simulink model "IPMSM_velocity_control"  (R2020b)
settings: Solver=FixedStepDiscrete  StartTime=0.0  StopTime=300e-3  FixedStep=Ts  RelTol=1e-3
PreLoadFcn:
  | ee_ipmsm_torque_based_load_control_data;
StopFcn:
  | ee_addSimlogTimeStamp(bdroot)
values from neighbouring files (symbols this model uses):
  K_aw = 100    [ee_ipmsm_torque_based_load_control_data.m]
  K_i = 200    [ee_ipmsm_torque_based_load_control_data.m]
  K_p = 1    [ee_ipmsm_torque_based_load_control_data.m]
  K_v = 1    [ee_ipmsm_torque_based_load_control_data.m]
  Ld = 0.00024368    [ee_ipmsm_torque_based_load_control_data.m]
  Lq = 0.00029758    [ee_ipmsm_torque_based_load_control_data.m]
  msg_period = 10e-3    (= 0.01)    [ee_ipmsm_torque_based_load_control_data.m]
  p = 5    [ee_ipmsm_torque_based_load_control_data.m]
  psim = 0.04366    [ee_ipmsm_torque_based_load_control_data.m]
  Ts = 5e-6    (= 5e-06)    [ee_ipmsm_torque_based_load_control_data.m]
undefined symbols (not defined in the file or in its folder): DiscIntNeverNeededParam, m, n, VDC_VECT
libraries: fl_lib x12, nesl_utility x12, ee_lib x5, fl_ps_legacy_lib x4, simulink x2, eeTransforms x2, slrealtimeutilitieslib x2, slrealtimeiplib x2, eePmsmCurrentController x1, eePmsmCurrentReferenceGen x1, eePmsmTorqueEstimator x1, eePwmGeneratorTwoLevel x1
CloseFcn:
  | try,close(h1_ee_ipmsm_torque_based_load_control),end
  | clear h1_ee_ipmsm_torque_based_load_control
  | 
  | clear simlog_ee_ipmsm_torque_based_load_control
  | clear logsout_ee_ipmsm_torque_based_load_control
Description:
  | IPMSM Torque-Based Load Control
settings Model: SimulationMode=accelerator  Creator=The MathWorks, Inc.  LastModifiedBy=Cliente
settings DataIOCC: MaxDataPoints=210000  ReturnWorkspaceOutputs=off  SignalLoggingName=logsout_ee_ipmsm_torque_based_load_control
settings OptimizationCC: DefaultParameterBehavior=Inlined  EnhancedBackFolding=on  PassReuseOutputArgsAs=Individual arguments  ZeroExternalMemoryAtStartup=off  ZeroInternalMemoryAtStartup=off  OptimizeBlockOrder=speed  DifferentSizesBufferReuse=on  OptimizationCustomize=off  EfficientTunableParamExpr=on
settings DebuggingCC: UnderspecifiedInitializationDetection=Classic  MergeDetectMultiDrivingBlocksExec=none  ParameterTunabilityLossMsg=error  SFUnexpectedBacktrackingDiag=warning  SFNoUnconditionalDefaultTransitionDiag=warning  SFExecutionAtInitializationDiag=none  ArithmeticOperatorsInVariantConditions=warning
settings SFSimCC: SimUseLocalCustomCode=off  MATLABDynamicMemAlloc=off  CustomCodeUndefinedFunction=UseInterfaceOnly
settings RTWCC: Description=Embedded Coder  SystemTargetFile=ert.tlc  TemplateMakefile=ert_default_tmf  RTWUseLocalCustomCode=off
settings CodeAppCC: ForceParamTrailComments=on  IgnoreCustomStorageClasses=off  OperatorAnnotations=on  SimulinkDataObjDesc=on  SFDataObjDesc=on  InsertBlockDesc=on
settings ERTTargetCC: GenerateSampleERTMain=on  InlinedParameterPlacement=NonHierarchical  ERTCustomFileTemplate=example_file_process.tlc
settings ConfigComp: CovMetricSettings=dw  CovSaveCumulativeToWorkspaceVar=on  CovSaveSingleToWorkspaceVar=on  CovExternalEMLEnable=off
settings SimscapeCC: SimscapeNormalizeSystem=off  SimscapeLogSimulationStatistics=on  SimscapeLogName=simlog_ee_ipmsm_torque_based_load_control  SimscapeLogDataHistory=210000

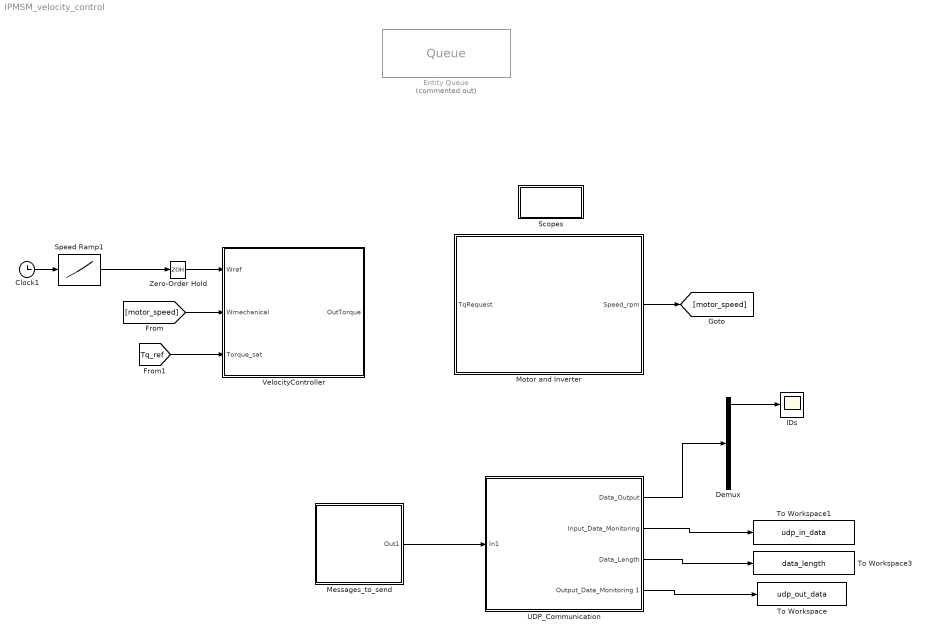
== system IPMSM_velocity_control ==
  Clock1 : Clock
  Demux : Demux  Outputs=5
  Entity Queue : Queue  Commented=on  InputPortMessageModes=m  OutputPortMessageModes=n,m  AverageWait=on
      settings: OutputPortMap=o2,o5
  IDs : Scope
  Messages_to_send : Subsystem
  Motor and Inverter : Subsystem
  Scopes : Subsystem
  Speed Ramp1 : Lookup_n-D  NumberOfTableDimensions=1  BreakpointsForDimension1=[0 .2 2]  Table=[0 200 200]  InternalRulePriority=Speed  RndMeth=Simplest  InputSameDT=on
  To Workspace : ToWorkspace  VariableName=udp_out_data  SaveFormat=Timeseries  SampleTime=-1
      settings: Save2DSignal=2-D array (concatenate along first dimension)
  To Workspace1 : ToWorkspace  VariableName=udp_in_data  SaveFormat=Timeseries  SampleTime=-1
      settings: Save2DSignal=2-D array (concatenate along first dimension)
  To Workspace3 : ToWorkspace  VariableName=data_length  SaveFormat=Timeseries  SampleTime=-1
      settings: Save2DSignal=2-D array (concatenate along first dimension)
  UDP_Communication : Subsystem
  VelocityController : Subsystem
  Zero-Order Hold : ZeroOrderHold  SampleTime=10e-3
  wires:
  Motor and Inverter/1(Speed_rpm) -> [motor_speed]
  Clock1/1 -> Speed Ramp1/1
  [Tq_ref] -> VelocityController/3(Torque_sat)
  Zero-Order Hold/1 -> VelocityController/1(Wref)
  Speed Ramp1/1 -> Zero-Order Hold/1
  Demux/1 -> IDs/1
  UDP_Communication/4(Output_Data_Monitoring 1) -> To Workspace/1
  UDP_Communication/2("Input_Data_Monitoring ") -> To Workspace1/1
  UDP_Communication/3(Data_Length) -> To Workspace3/1
  UDP_Communication/1(Data_Output) -> Demux/1
  Messages_to_send/1(Out1) -> UDP_Communication/1(In1)
  [motor_speed] -> VelocityController/2(Wmechanical)

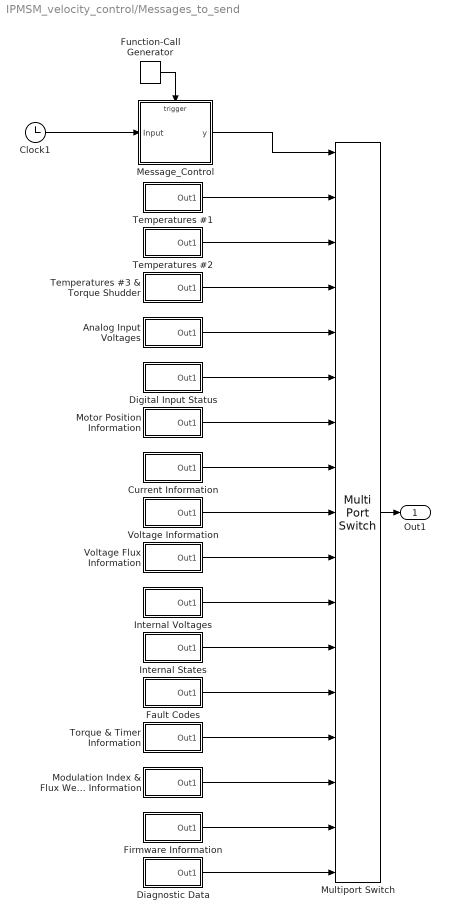
== system IPMSM_velocity_control/Messages_to_send ==
  Analog Input Voltages : Subsystem
  Clock1 : Clock
  Current Information : Subsystem
  Diagnostic Data : Subsystem
  Digital Input Status : Subsystem
  Fault Codes : Subsystem
  Firmware Information : Subsystem
  Function-Call Generator : simulink/Ports & Subsystems/Function-Call Generator  sample_time=1e-5  numberOfIterations=1  DisallowWideOutput=off
  Internal States : Subsystem
  Internal Voltages : Subsystem
  Message_Control : Subsystem
  Modulation Index & Flux Weakening Output Information : Subsystem
  Motor Position Information : Subsystem
  Multiport Switch : MultiPortSwitch  Inputs=16  DiagnosticForDefault=None
  Temperatures #1 : Subsystem
  Temperatures #2 : Subsystem
  Temperatures #3 & Torque Shudder : Subsystem
  Torque & Timer Information : Subsystem
  Voltage Flux Information : Subsystem
  Voltage Information : Subsystem
  Out1 : Outport
  wires:
  Function-Call Generator/1 -> Message_Control/Trigger
  Diagnostic Data/1(Out1) -> Multiport Switch/17
  Voltage Information/1(Out1) -> Multiport Switch/9
  Clock1/1 -> Message_Control/1(Input)
  Message_Control/1(y) -> Multiport Switch/1
  Digital Input Status/1(Out1) -> Multiport Switch/6
  Voltage Flux Information/1(Out1) -> Multiport Switch/10
  Internal Voltages/1(Out1) -> Multiport Switch/11
  Current Information/1(Out1) -> Multiport Switch/8
  Fault Codes/1(Out1) -> Multiport Switch/13
  Torque & Timer Information/1(Out1) -> Multiport Switch/14
  Internal States/1(Out1) -> Multiport Switch/12
  Firmware Information/1(Out1) -> Multiport Switch/16
  Modulation Index & Flux Weakening Output Information/1(Out1) -> Multiport Switch/15
  Multiport Switch/1 -> Out1/1
  Temperatures #2/1(Out1) -> Multiport Switch/3
  Temperatures #3 & Torque Shudder/1(Out1) -> Multiport Switch/4
  Analog Input Voltages/1(Out1) -> Multiport Switch/5
  Motor Position Information/1(Out1) -> Multiport Switch/7
  Temperatures #1/1(Out1) -> Multiport Switch/2

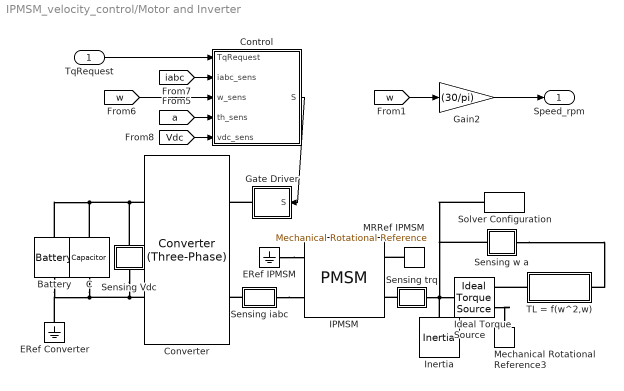
== system IPMSM_velocity_control/Motor and Inverter ==
  TqRequest : Inport
  Battery : ee_lib/Sources/Battery  Vnom=Vnom V  prm_dir=1  R1_dis=2 Ohm  R1_ch=2 Ohm  R1=0.001 Ohm  prm_AH=1  AH=10000 hr*A  V1=V1 V  AH1=3000 hr*A  prm_R2=1  R2=2000 Ohm  prm_dyn=1  Rp1=0.005 Ohm  tau1=30 s  Rp2=0.005 Ohm  tau2=30 s  Rp3=0.005 Ohm  tau3=30 s  Rp4=0.005 Ohm  tau4=30 s  Rp5=0.005 Ohm  tau5=30 s  prm_fade=1  N_fade=100  AH_fade=45 hr*A  R1_fade=2.02 Ohm  R1_ch_fade=2.02 Ohm  V1_fade=10.35 V  i_specify=off  i_priority=None  i=0 A  i_nominal_specify=off  i_nominal_unit=A  i_nominal_value=1  v_specify=off  v_priority=None  v=0 V  v_nominal_specify=off  v_nominal_unit=V  v_nominal_value=1  charge_specify=on  charge_priority=High  charge=8000 hr*A  charge_nominal_specify=off  charge_nominal_unit=hr*A  charge_nominal_value=1  num_cycles_specify=off  num_cycles_priority=High  num_cycles=0  num_cycles_nominal_specify=off  num_cycles_nominal_unit=1  num_cycles_nominal_value=1  thermal_mass=30000 J/K  Tmeas=298.15 K  Vnom_T2=12 V  R1_T2=2.2 Ohm  R1_T2_dis=2.2 Ohm  R1_T2_ch=2.2 Ohm  V1_T2=11.4 V  R2_T2=2200 Ohm  Rp1_T2=0.005 Ohm  tau1_T2=30 s  Rp2_T2=0.005 Ohm  tau2_T2=30 s  Rp3_T2=0.005 Ohm  tau3_T2=30 s  Rp4_T2=0.005 Ohm  tau4_T2=30 s  Rp5_T2=0.005 Ohm  tau5_T2=30 s  Tmeas2=273.15 K  temperature_specify=off  temperature_priority=High  temperature=298.15 K  temperature_nominal_specify=off  temperature_nominal_unit=K  temperature_nominal_value=1
      settings: SourceProductName=Electrical
  C : fl_lib/Electrical/Electrical Elements/Capacitor  c=Cdc F  r=1e-6 Ohm  g=0 1/Ohm  i_specify=off  i_priority=None  i=0 A  i_nominal_specify=off  i_nominal_unit=A  i_nominal_value=1  v_specify=off  v_priority=None  v=0 V  v_nominal_specify=off  v_nominal_unit=V  v_nominal_value=1  vc_specify=on  vc_priority=None  vc=Vnom V  vc_nominal_specify=off  vc_nominal_unit=V  vc_nominal_value=1
      settings: SourceProductName=Foundation Library
  Control : Subsystem
  Converter : ee_lib/Semiconductors & Converters/Converters/Converter (Three-Phase)  device_type=3  Vf=0.8 V  Ron=0.001 Ohm  Rds=0.001 Ohm  Goff=1e-5 1/Ohm  Vth=0.5 V  Vgt=1 V  Vgt_off=-1 V  Ih=1 A  diode_param=2  diode_Vf=0.8 V  diode_Ron=0.001 Ohm  diode_Goff=1e-5 1/Ohm  diode_C=50 nF  diode_iRM=-235 A  diode_iF=300 A  diode_idot=-50 A/us  diode_trr_param=1  diode_trr_factor=3  diode_trr=15 us  diode_Qrr=1.5e+3 s*uA  snubber_type=0  Rs=0.1 Ohm  Cs=1e-7 F
      settings: SourceProductName=Electrical
  ERef Converter : fl_lib/Electrical/Electrical Elements/Electrical Reference
      settings: SourceProductName=Foundation Library
  ERef IPMSM : fl_lib/Electrical/Electrical Elements/Electrical Reference
      settings: SourceProductName=Foundation Library
  Gain2 : Gain  Gain=(30/pi)
  Gate Driver : Subsystem
  IPMSM : ee_lib/Electromechanical/Permanent Magnet/PMSM  winding_type=ee.enum.statorconnection.wye  machine_param=ee.enum.pmsm.parameterization.constant  nPolePairs=p  pmflux_param=ee.enum.pmflux.fluxlinkage  pm_flux_linkage=psim Wb  torque_constant=0.18 N*m/A  back_emf_constant=0.18 V/(rad/s)  stator_param=ee.enum.statorparam.LdLqL0  Ld=Ld H  Lq=Lq H  idVec=[-200, 0, 200] A  iqVec=[-200, 0, 200] A  LdMatrix=0.0002 * ones(3, 3) H  LqMatrix=0.0002 * ones(3, 3) H  PmMatrix=0.1 * ones(3, 3) Wb  ktMatrix=0.18 * ones(3, 3) N*m/A  keMatrix=0.18 * ones(3, 3) V/(rad/s)  L0=L0 H  Ls=0.0002 H  Lm=0.00002 H  Ms=0.00002 H  Rs=Rs Ohm  zero_sequence=ee.enum.park.zerosequence.exclude  J=0 kg*m^2  lam=0 N*m/(rad/s)  axes_param=ee.enum.rotorangle.qaxis  i_d_specify=off  i_d_priority=None  i_d=0 A  i_d_nominal_specify=off  i_d_nominal_unit=A  i_d_nominal_value=1  i_q_specify=off  i_q_priority=None  i_q=0 A  i_q_nominal_specify=off  i_q_nominal_unit=A  i_q_nominal_value=1  torque_specify=off  torque_priority=None  torque=0 N*m  torque_nominal_specify=off  torque_nominal_unit=N*m  torque_nominal_value=1  angular_velocity_specify=on  angular_velocity_priority=None  angular_velocity=0 rpm  angular_velocity_nominal_specify=off  angular_velocity_nominal_unit=rpm  angular_velocity_nominal_value=1  angular_position_specify=off  angular_position_priority=None  angular_position=0 deg  angular_position_nominal_specify=off  angular_position_nominal_unit=deg  angular_position_nominal_value=1  loss_param=ee.enum.ironloss.none  losses_oc=[0, 0, 0] W  losses_sc=[0, 0, 0] W  f_losses=60 Hz  Isc_losses=95 A  Tmeas=298.15 K  alpha=3.93e-3 1/K  alpha_flux=-0.001 1/K  stator_thermal_mass=100 J/K  rotor_thermal_mass=200 J/K  Rm_percent_rotor=90  Rd_percent_rotor=30  temperatureA_specify=off  temperatureA_priority=High  temperatureA=25 degC  temperatureA_nominal_specify=off  temperatureA_nominal_unit=degC  temperatureA_nominal_value=1  temperatureB_specify=off  temperatureB_priority=High  temperatureB=25 degC  temperatureB_nominal_specify=off  temperatureB_nominal_unit=degC  temperatureB_nominal_value=1  temperatureC_specify=off  temperatureC_priority=High  temperatureC=25 degC  temperatureC_nominal_specify=off  temperatureC_nominal_unit=degC  temperatureC_nominal_value=1  temperatureR_specify=off  temperatureR_priority=High  temperatureR=25 degC  temperatureR_nominal_specify=off  temperatureR_nominal_unit=degC  temperatureR_nominal_value=1
      settings: AttributesFormatString=35 kW  SourceProductName=Electrical  InternalSimscapePortConfiguration="{\"Bottom\":[],\"Left\":[{\"id\":\"N\",\"label\":\"~\",\"type\":\"foundation.electrical.three_phase\"},{\"id\":\"n\",\"label\":\"n\",\"type\":\"foundation.electrical.electrical\"}],\"Right\":[{\"id\":\"R\",\"label\":\"R\",\"type\":\"foundation.mechanical.rotational.rotational\"},{\"id\":\"C\",\"label\":\"C\",\"type\":\"foundation.mechanical.rotational.rotational\"}],\"Top\":[]}"
  Ideal Torque Source : fl_lib/Mechanical/Mechanical Sources/Ideal Torque Source
      settings: SourceProductName=Foundation Library
  Inertia : fl_lib/Mechanical/Rotational Elements/Inertia  inertia=Jm kg*m^2  num_ports=foundation.enum.numPorts2.one  w_specify=off  w_priority=High  w=0 rad/s  w_nominal_specify=off  w_nominal_unit=rad/s  w_nominal_value=1  t_specify=off  t_priority=None  t=0 N*m  t_nominal_specify=off  t_nominal_unit=N*m  t_nominal_value=1
      settings: SourceProductName=Foundation Library
  MRRef IPMSM : fl_lib/Mechanical/Rotational Elements/Mechanical Rotational Reference
      settings: SourceProductName=Foundation Library
  Mechanical Rotational Reference3 : fl_lib/Mechanical/Rotational Elements/Mechanical Rotational Reference
      settings: SourceProductName=Foundation Library
  Sensing Vdc : Subsystem
      mask Display: disp('vdc')
  Sensing trq : Subsystem
      mask Display: disp('trq')
  Sensing w a : Subsystem
      mask Display: disp('w,a')
  Sensing iabc : Subsystem
      mask Display: disp('iabc')
  Solver Configuration : nesl_utility/Solver Configuration  PhysicalDomain=network_engine_domain  SubClassName=solver  LeftPortType=input  RightPortType=generic  Tones=[]  Harmonics=[]  SimulateNoise=off  Profile=off  UseLocalSampling=off  EnableSwitchedLinearOptims=on  FrequencyDomain=off  UseCCode=off  RelTol=0.001  AbsTol=1e-06  MinStep=1e-09  ToWorkspace=off  RevertToSquareIcSolve=off  NumHomotopyIterations=100  PhasorMode=off  PhasorModeNumHarmonics=1  DoDC=off  ResidualTolerance=1e-9  UseLocalSolver=on  LocalSolverChoice=NE_BACKWARD_EULER_ADVANCER  LocalSolverSampleTime=Ts  DoFixedCost=on  MaxNonlinIter=5  MaxModeIter=2  ComputeImpulses=off  ImpulseIterations=2  LinearAlgebra=auto  EquationFormulation=NE_TIME_EF  DelaysMemoryBudget=1024  AutomaticFiltering=on  FilteringTimeConstant=0.001  PartitionStorageMethod=AS_NEEDED  PartitionMemoryBudget=1024  PartitionMethod=FAST
      settings: SourceProductName=Utilities
  TL = f(w^2,w) : Subsystem
  Speed_rpm : Outport
  wires:
  [w] -> Control/3(w_sens)
  [iabc] -> Control/2(iabc_sens)
  [a] -> Control/4(th_sens)
  [Vdc] -> Control/5(vdc_sens)
  TqRequest/1 -> Control/1(TqRequest)
  [w] -> Gain2/1
  Gain2/1 -> Speed_rpm/1
  Control/1(S) -> Gate Driver/1(S)
  connections:
  MRRef IPMSM/LConn1 -- IPMSM/RConn2
  Ideal Torque Source/RConn2 -- Mechanical Rotational Reference3/LConn1
  Converter/RConn2 -- Battery/RConn1 -- ERef Converter/LConn1 -- C/RConn1 -- Sensing Vdc/RConn1
  ERef IPMSM/LConn1 -- IPMSM/LConn2
  Gate Driver/RConn1 -- Converter/LConn1
  Sensing iabc/LConn1 -- Converter/LConn2
  Converter/RConn1 -- Battery/LConn1 -- C/LConn1 -- Sensing Vdc/LConn1
  Sensing w a/RConn1 -- TL = f(w^2,w)/LConn1
  Sensing trq/RConn1 -- Sensing w a/LConn1 -- Solver Configuration/RConn1 -- Ideal Torque Source/LConn1 -- Inertia/LConn1
  Sensing iabc/RConn1 -- IPMSM/LConn1
  TL = f(w^2,w)/RConn1 -- Ideal Torque Source/RConn1
  Sensing trq/LConn1 -- IPMSM/RConn1

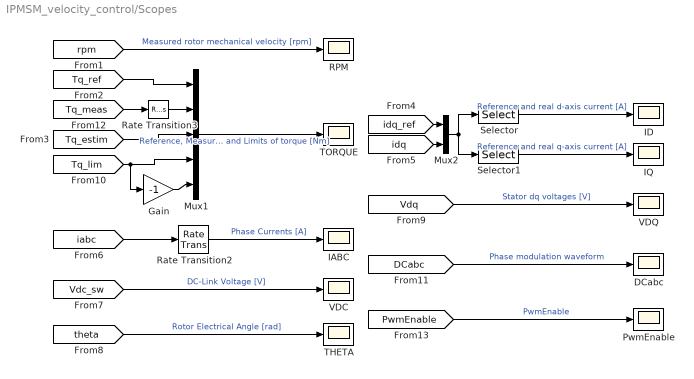
== system IPMSM_velocity_control/Scopes ==
  DCabc : Scope
  Gain : Gain  Gain=-1
  IABC : Scope
  ID : Scope
  IQ : Scope
  Mux1 : Mux  Inputs=5
  Mux2 : Mux  Inputs=2
  PwmEnable : Scope
  RPM : Scope
  Rate Transition2 : RateTransition  OutPortSampleTime=1e-4
  Rate Transition3 : RateTransition
  Selector : Selector  InputPortWidth=4  IndexOptions=Index vector (dialog)  Indices=[1 3]  OutputSizes=1
  Selector1 : Selector  InputPortWidth=4  IndexOptions=Index vector (dialog)  Indices=[2 4]  OutputSizes=1
  THETA : Scope
  TORQUE : Scope
  VDC : Scope
  VDQ : Scope
  wires:
  [rpm] -> RPM/1  "Measured rotor mechanical velocity [rpm]"
  Mux1/1 -> TORQUE/1  "Reference, Measured, Estim and Limits of torque [Nm]"
  [Tq_ref] -> Mux1/1
  [iabc] -> Rate Transition2/1
  [theta] -> THETA/1  "Rotor Electrical Angle [rad]"
  [Vdq] -> VDQ/1  "Stator dq voltages [V]"
  [DCabc] -> DCabc/1  "Phase modulation waveform"
  [Vdc_sw] -> VDC/1  "DC-Link Voltage [V]"
  Rate Transition2/1 -> IABC/1  "Phase Currents [A]"
  Selector1/1 -> IQ/1  "Reference and real q-axis current [A]"
  [idq_ref] -> Mux2/1
  Selector/1 -> ID/1  "Reference and real d-axis current [A]"
  Mux2/1 -> Selector1/1, Selector/1
  [idq] -> Mux2/2
  [Tq_estim] -> Mux1/3
  [Tq_meas] -> Rate Transition3/1
  Rate Transition3/1 -> Mux1/2
  [PwmEnable] -> PwmEnable/1  "PwmEnable"
  [Tq_lim] -> Mux1/4, Gain/1
  Gain/1 -> Mux1/5

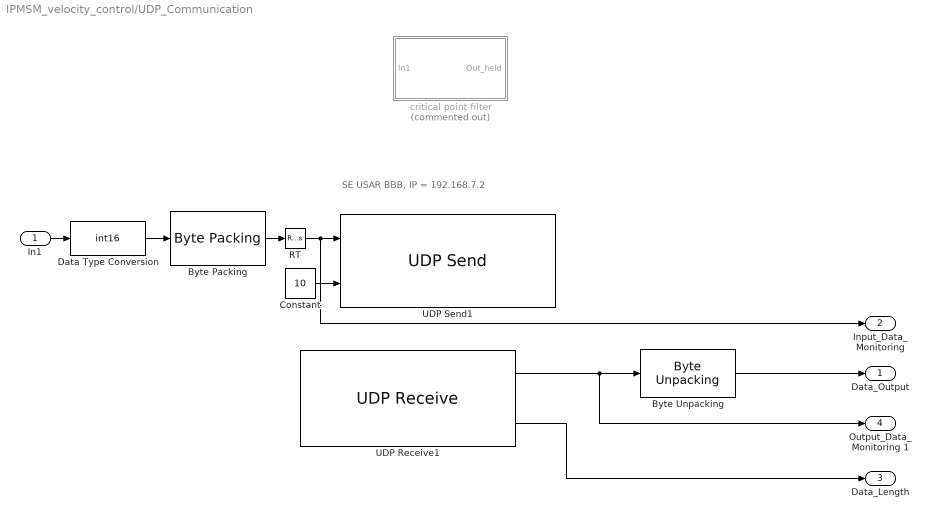
== system IPMSM_velocity_control/UDP_Communication ==
  note: SE USAR BBB, IP = 192.168.7.2
  In1 : Inport
  Byte Packing : slrealtimeutilitieslib/Byte Packing  MaskPackedDataType=uint8  MaskUnpackedDataTypes={'int16'}  MaskAlignment=1
  Byte Unpacking : slrealtimeutilitieslib/Byte Unpacking  MaskUnpackedDataTypes={'int16'}  MaskUnpackedDataSizes={[5]}  MaskAlignment=1
      settings: SourceProductBaseCode=XP
  Constant : Constant  Value=10
  Data Type Conversion : DataTypeConversion  OutDataTypeStr=int16
  RT : RateTransition
  UDP Receive1 : slrealtimeiplib/UDP Receive  useHostTargetConn=on  ipAddress=127.0.0.1  localPort=8082  rcvWidth=10  rcvFmAny=off  fmAddress=127.0.0.1  rcvMulticast=off  multicastAddress={}  sampleTime=0.5e-4
      settings: SourceProductBaseCode=XP
  UDP Send1 : slrealtimeiplib/UDP Send  useHostTargetConn=on  ipAddress=127.0.0.1  localPort=8080  toAddress=127.0.0.1  toPort=8082  sampleTime=1e-3
      settings: SourceProductBaseCode=XP
  "critical point filter " : Subsystem  Commented=on
  Data_Output : Outport
  "Input_Data_Monitoring " : Outport  Port=2
  Data_Length : Outport  Port=3
  Output_Data_Monitoring 1 : Outport  Port=4
  wires:
  In1/1 -> Data Type Conversion/1
  Data Type Conversion/1 -> Byte Packing/1
  UDP Receive1/1 -> Output_Data_Monitoring 1/1, Byte Unpacking/1
  Constant/1 -> UDP Send1/2
  Byte Packing/1 -> RT/1
  RT/1 -> "Input_Data_Monitoring "/1, UDP Send1/1
  UDP Receive1/2 -> Data_Length/1
  Byte Unpacking/1 -> Data_Output/1

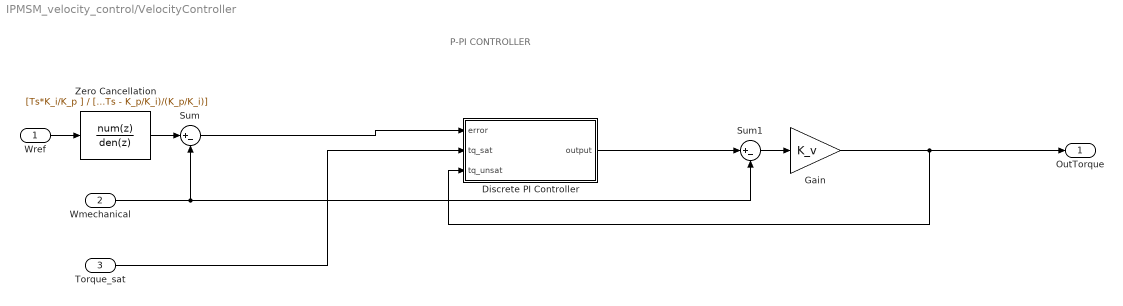
== system IPMSM_velocity_control/VelocityController ==
  note: P-PI CONTROLLER
  Wref : Inport
  Wmechanical : Inport  Port=2
  Torque_sat : Inport  Port=3
  Discrete PI Controller : Subsystem
  Gain : Gain  Gain=K_v
  Sum : Sum  Inputs=|+-
  Sum1 : Sum  Inputs=|+-
  Zero Cancellation : DiscreteTransferFcn  Numerator=[Ts*K_i/K_p ]  Denominator="[1  (Ts - K_p/K_i)/(K_p/K_i)]"  SampleTime=msg_period
  OutTorque : Outport
  wires:
  Sum1/1 -> Gain/1
  Wmechanical/1 -> Sum1/2, Sum/2
  Sum/1 -> Discrete PI Controller/1(error)
  Gain/1 -> Discrete PI Controller/3(tq_unsat), OutTorque/1
  Torque_sat/1 -> Discrete PI Controller/2(tq_sat)
  Wref/1 -> Zero Cancellation/1
  Zero Cancellation/1 -> Sum/1
  Discrete PI Controller/1(output) -> Sum1/1

== system IPMSM_velocity_control/Messages_to_send/Analog Input Voltages ==
  Constant3 : Constant  Value=168
  Mux : Mux  Inputs=5
  Sine Wave{,1..3} (4 alike) : Sin  Amplitude=100  SampleTime=0
  Out1 : Outport
  wires:
  Mux/1 -> Out1/1
  Constant3/1 -> Mux/1
  Sine Wave3/1 -> Mux/5
  Sine Wave1/1 -> Mux/3
  Sine Wave2/1 -> Mux/4
  Sine Wave/1 -> Mux/2

== system IPMSM_velocity_control/Messages_to_send/Current Information ==
  Constant2 : Constant  Value=171
  Mux : Mux  Inputs=5
  Sine Wave{,1..3} (4 alike) : Sin  Amplitude=100  SampleTime=0
  Out1 : Outport
  wires:
  Mux/1 -> Out1/1
  Constant2/1 -> Mux/1
  Sine Wave3/1 -> Mux/5
  Sine Wave2/1 -> Mux/4
  Sine Wave/1 -> Mux/2
  Sine Wave1/1 -> Mux/3

== system IPMSM_velocity_control/Messages_to_send/Diagnostic Data ==
  Constant2 : Constant  Value=180
  Mux : Mux  Inputs=5
  Sine Wave{,1..3} (4 alike) : Sin  Amplitude=100  SampleTime=0
  Out1 : Outport
  wires:
  Mux/1 -> Out1/1
  Constant2/1 -> Mux/1
  Sine Wave2/1 -> Mux/4
  Sine Wave1/1 -> Mux/3
  Sine Wave3/1 -> Mux/5
  Sine Wave/1 -> Mux/2

== system IPMSM_velocity_control/Messages_to_send/Digital Input Status ==
  Constant2 : Constant  Value=169
  Mux : Mux  Inputs=5
  Sine Wave{,1..3} (4 alike) : Sin  Amplitude=100  SampleTime=0
  Out1 : Outport
  wires:
  Mux/1 -> Out1/1
  Constant2/1 -> Mux/1
  Sine Wave3/1 -> Mux/5
  Sine Wave2/1 -> Mux/4
  Sine Wave/1 -> Mux/2
  Sine Wave1/1 -> Mux/3

== system IPMSM_velocity_control/Messages_to_send/Fault Codes ==
  Constant2 : Constant  Value=176
  Mux : Mux  Inputs=5
  Sine Wave{,1..3} (4 alike) : Sin  Amplitude=100  SampleTime=0
  Out1 : Outport
  wires:
  Mux/1 -> Out1/1
  Constant2/1 -> Mux/1
  Sine Wave2/1 -> Mux/4
  Sine Wave1/1 -> Mux/3
  Sine Wave3/1 -> Mux/5
  Sine Wave/1 -> Mux/2

== system IPMSM_velocity_control/Messages_to_send/Firmware Information ==
  Constant2 : Constant  Value=179
  Mux : Mux  Inputs=5
  Sine Wave{,1..3} (4 alike) : Sin  Amplitude=100  SampleTime=0
  Out1 : Outport
  wires:
  Constant2/1 -> Mux/1
  Mux/1 -> Out1/1
  Sine Wave2/1 -> Mux/4
  Sine Wave1/1 -> Mux/3
  Sine Wave3/1 -> Mux/5
  Sine Wave/1 -> Mux/2

== system IPMSM_velocity_control/Messages_to_send/Internal States ==
  Constant2 : Constant  Value=175
  Mux : Mux  Inputs=5
  Sine Wave{,1..3} (4 alike) : Sin  Amplitude=100  SampleTime=0
  Out1 : Outport
  wires:
  Mux/1 -> Out1/1
  Constant2/1 -> Mux/1
  Sine Wave2/1 -> Mux/4
  Sine Wave1/1 -> Mux/3
  Sine Wave3/1 -> Mux/5
  Sine Wave/1 -> Mux/2

== system IPMSM_velocity_control/Messages_to_send/Internal Voltages ==
  Constant2 : Constant  Value=174
  Mux : Mux  Inputs=5
  Sine Wave{,1..3} (4 alike) : Sin  Amplitude=100  SampleTime=0
  Out1 : Outport
  wires:
  Mux/1 -> Out1/1
  Constant2/1 -> Mux/1
  Sine Wave2/1 -> Mux/4
  Sine Wave1/1 -> Mux/3
  Sine Wave3/1 -> Mux/5
  Sine Wave/1 -> Mux/2

== system IPMSM_velocity_control/Messages_to_send/Message_Control ==
  Input : Inport
  Trigger : TriggerPort  TriggerType=function-call  VariantControl=Variant  PortDimensions=1
  MATLAB Function : MATLAB Function  TreatAsAtomicUnit=on
  y : Outport
  wires:
  MATLAB Function/1(y) -> y/1
  Input/1 -> MATLAB Function/1(u)

== system IPMSM_velocity_control/Messages_to_send/Modulation Index & Flux Weakening Output Information ==
  Constant2 : Constant  Value=178
  Mux : Mux  Inputs=5
  Sine Wave{,1..3} (4 alike) : Sin  Amplitude=100  SampleTime=0
  Out1 : Outport
  wires:
  Mux/1 -> Out1/1
  Constant2/1 -> Mux/1
  Sine Wave2/1 -> Mux/4
  Sine Wave1/1 -> Mux/3
  Sine Wave3/1 -> Mux/5
  Sine Wave/1 -> Mux/2

== system IPMSM_velocity_control/Messages_to_send/Motor Position Information ==
  Constant2 : Constant  Value=170
  Mux : Mux  Inputs=5
  Sine Wave{,1..3} (4 alike) : Sin  Amplitude=100  SampleTime=0
  Out1 : Outport
  wires:
  Constant2/1 -> Mux/1
  Mux/1 -> Out1/1
  Sine Wave3/1 -> Mux/5
  Sine Wave2/1 -> Mux/4
  Sine Wave/1 -> Mux/2
  Sine Wave1/1 -> Mux/3

== system IPMSM_velocity_control/Messages_to_send/Temperatures #1 ==
  Constant3 : Constant  Value=165
  Mux : Mux  Inputs=5
  Sine Wave{,1..3} (4 alike) : Sin  Amplitude=100  SampleTime=0
  Out1 : Outport
  wires:
  Mux/1 -> Out1/1
  Sine Wave/1 -> Mux/2
  Constant3/1 -> Mux/1
  Sine Wave1/1 -> Mux/3
  Sine Wave2/1 -> Mux/4
  Sine Wave3/1 -> Mux/5

== system IPMSM_velocity_control/Messages_to_send/Temperatures #2 ==
  Constant3 : Constant  Value=166
  Mux : Mux  Inputs=5
  Sine Wave{,1..3} (4 alike) : Sin  Amplitude=100  SampleTime=0
  Out1 : Outport
  wires:
  Mux/1 -> Out1/1
  Constant3/1 -> Mux/1
  Sine Wave3/1 -> Mux/5
  Sine Wave1/1 -> Mux/3
  Sine Wave2/1 -> Mux/4
  Sine Wave/1 -> Mux/2

== system IPMSM_velocity_control/Messages_to_send/Temperatures #3 & Torque Shudder ==
  Constant3 : Constant  Value=167
  Mux : Mux  Inputs=5
  Sine Wave{,1..3} (4 alike) : Sin  Amplitude=100  SampleTime=0
  Out1 : Outport
  wires:
  Mux/1 -> Out1/1
  Constant3/1 -> Mux/1
  Sine Wave3/1 -> Mux/5
  Sine Wave1/1 -> Mux/3
  Sine Wave2/1 -> Mux/4
  Sine Wave/1 -> Mux/2

== system IPMSM_velocity_control/Messages_to_send/Torque & Timer Information ==
  Constant2 : Constant  Value=177
  Mux : Mux  Inputs=5
  Sine Wave{,1..3} (4 alike) : Sin  Amplitude=100  SampleTime=0
  Out1 : Outport
  wires:
  Constant2/1 -> Mux/1
  Mux/1 -> Out1/1
  Sine Wave2/1 -> Mux/4
  Sine Wave1/1 -> Mux/3
  Sine Wave3/1 -> Mux/5
  Sine Wave/1 -> Mux/2

== system IPMSM_velocity_control/Messages_to_send/Voltage Flux Information ==
  Constant2 : Constant  Value=173
  Mux : Mux  Inputs=5
  Sine Wave{,1..3} (4 alike) : Sin  Amplitude=100  SampleTime=0
  Out1 : Outport
  wires:
  Mux/1 -> Out1/1
  Constant2/1 -> Mux/1
  Sine Wave2/1 -> Mux/4
  Sine Wave1/1 -> Mux/3
  Sine Wave3/1 -> Mux/5
  Sine Wave/1 -> Mux/2

== system IPMSM_velocity_control/Messages_to_send/Voltage Information ==
  Constant2 : Constant  Value=172
  Mux : Mux  Inputs=5
  Sine Wave{,1..3} (4 alike) : Sin  Amplitude=100  SampleTime=0
  Out1 : Outport
  wires:
  Mux/1 -> Out1/1
  Constant2/1 -> Mux/1
  Sine Wave2/1 -> Mux/4
  Sine Wave1/1 -> Mux/3
  Sine Wave3/1 -> Mux/5
  Sine Wave/1 -> Mux/2

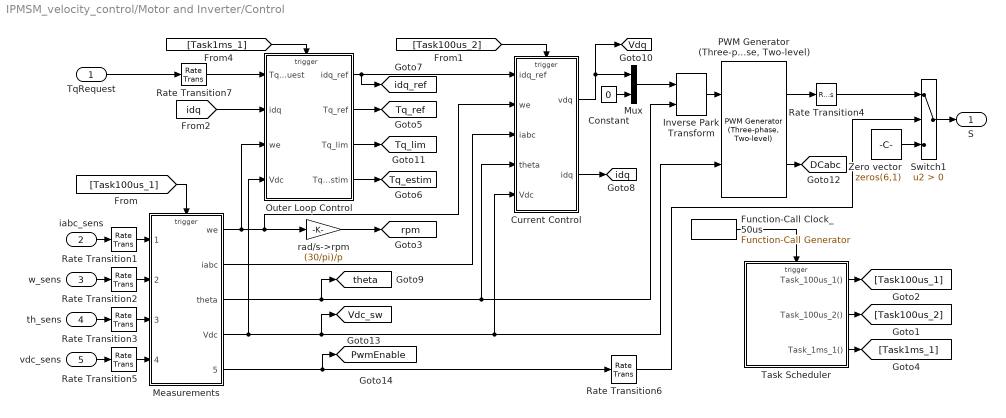
== system IPMSM_velocity_control/Motor and Inverter/Control ==
  TqRequest : Inport
  iabc_sens : Inport  Port=2
  w_sens : Inport  Port=3
  th_sens : Inport  Port=4
  vdc_sens : Inport  Port=5
  Constant : Constant  Value=0  SampleTime=-1
  Current Control : Subsystem
  Function-Call Clock_50us : simulink/Ports & Subsystems/Function-Call Generator  sample_time=5e-5  numberOfIterations=1  DisallowWideOutput=off
  Inverse Park Transform : eeTransforms/Inverse Park Transform  AxisAlignment=Q-axis  PowerInvariant=off
  Measurements : Subsystem
  Mux : Mux  Inputs=2
  Outer Loop Control : Subsystem
  "PWM Generator (Three-phase, Two-level)" : eePwmGeneratorTwoLevel/PWM Generator (Three-phase, Two-level)  PWMMode=Continuous PWM (CPWM)  CPWMMode=SVM: space vector modulation  DPWMMode=60 DPWM: 60 degree discontinuous PWM  fsw=fsw  Ts=Ts
      settings: SourceProductBaseCode=PS
  Rate Transition{1..7} (7 alike) : RateTransition
  Switch1 : Switch  Criteria=u2 > Threshold
  Task Scheduler : Stateflow chart  TreatAsAtomicUnit=on
  Zero vector : Constant  Value=zeros(6,1)
  rad/s->rpm : Gain  Gain=(30/pi)/p
  S : Outport  VectorParamsAs1DForOutWhenUnconnected=off
  tag scope: DCabc=global, PwmEnable=global, Tq_estim=global, Tq_lim=global, Tq_ref=global, Vdc_sw=global, Vdq=global, idq=global, idq_ref=global, rpm=global, theta=global
  wires:
  [Task100us_2] -> Current Control/Trigger
  [Task1ms_1] -> Outer Loop Control/Trigger
  Current Control/1(vdq) -> Mux/1, [Vdq]
  Measurements/2(iabc) -> Current Control/3(iabc)
  Measurements/3(theta) -> [theta], Inverse Park Transform/2, Current Control/4(theta)
  "PWM Generator (Three-phase, Two-level)"/1 -> Rate Transition4/1
  Inverse Park Transform/1 -> "PWM Generator (Three-phase, Two-level)"/1
  iabc_sens/1 -> Rate Transition1/1
  w_sens/1 -> Rate Transition2/1
  th_sens/1 -> Rate Transition3/1
  vdc_sens/1 -> Rate Transition5/1
  Outer Loop Control/1(idq_ref) -> Current Control/1(idq_ref), [idq_ref]
  "PWM Generator (Three-phase, Two-level)"/2 -> [DCabc]
  Rate Transition1/1 -> Measurements/1(iabc_sens)
  Rate Transition2/1 -> Measurements/2(w_sens)
  Rate Transition3/1 -> Measurements/3(th_sens)
  Rate Transition5/1 -> Measurements/4(Vdc_sens)
  Measurements/4(Vdc) -> Outer Loop Control/4(Vdc), [Vdc_sw], Current Control/5(Vdc), "PWM Generator (Three-phase, Two-level)"/2
  Function-Call Clock_50us/1 -> Task Scheduler/Trigger
  Task Scheduler/3(Task_1ms_1()) -> [Task1ms_1]
  Task Scheduler/2(Task_100us_2()) -> [Task100us_2]
  Task Scheduler/1(Task_100us_1()) -> [Task100us_1]
  Outer Loop Control/2(Tq_ref) -> [Tq_ref]
  Measurements/1(we) -> Outer Loop Control/3(we), Current Control/2(we), rad/s->rpm/1
  rad/s->rpm/1 -> [rpm]
  Outer Loop Control/3(Tq_lim) -> [Tq_lim]
  Rate Transition7/1 -> Outer Loop Control/1(TqRequest)
  TqRequest/1 -> Rate Transition7/1
  Outer Loop Control/4(Tq_estim) -> [Tq_estim]
  [idq] -> Outer Loop Control/2(idq)
  Switch1/1 -> S/1
  Rate Transition4/1 -> Switch1/1
  Measurements/5(PwmEnable) -> Rate Transition6/1, [PwmEnable]
  Zero vector/1 -> Switch1/3
  Rate Transition6/1 -> Switch1/2
  Current Control/2(idq) -> [idq]
  [Task100us_1] -> Measurements/Trigger
  Constant/1 -> Mux/2
  Mux/1 -> Inverse Park Transform/1

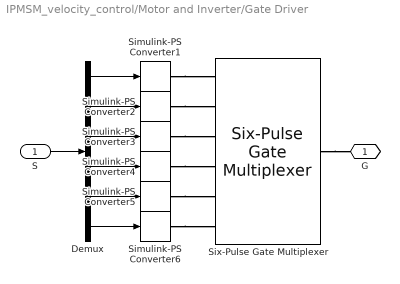
== system IPMSM_velocity_control/Motor and Inverter/Gate Driver ==
  S : Inport
  Demux : Demux  Outputs=6
  Simulink-PS Converter{1..6} (6 alike) : nesl_utility/Simulink-PS Converter  PhysicalDomain=network_engine_domain  SubClassName=ps_input  LeftPortType=input  RightPortType=output  PseudoPeriodic=off  Frequencies=[]  NoiseDistribution=none  NoiseParameters=[]  Unit=1  AffineConversion=off  FilteringAndDerivatives=zero  SimscapeFilterOrder=1  InputFilterTimeConstant=0.001  UdotUserProvided=1
      settings: SourceProductName=Utilities
  Six-Pulse Gate Multiplexer : ee_lib/Semiconductors & Converters/Converters/Six-Pulse Gate Multiplexer  R=0 Ohm
      settings: SourceProductName=Electrical  InternalSimscapePortConfiguration="{\"Bottom\":[],\"Left\":[{\"id\":\"GaH\",\"label\":\"Ga(H)\",\"type\":\"input\"},{\"id\":\"GaL\",\"label\":\"Ga(L)\",\"type\":\"input\"},{\"id\":\"GbH\",\"label\":\"Gb(H)\",\"type\":\"input\"},{\"id\":\"GbL\",\"label\":\"Gb(L)\",\"type\":\"input\"},{\"id\":\"GcH\",\"label\":\"Gc(H)\",\"type\":\"input\"},{\"id\":\"GcL\",\"label\":\"Gc(L)\",\"type\":\"input\"}],\"Right\":[{\"id\":\"p\",\"label\":\"G\",\"type\":\"foundation.electrical.twelve_phase\"}],\"Top\":[]}"
  G : PMIOPort  Side=Right
  wires:
  Demux/1 -> Simulink-PS Converter1/1
  S/1 -> Demux/1
  Demux/4 -> Simulink-PS Converter4/1
  Demux/2 -> Simulink-PS Converter2/1
  Demux/3 -> Simulink-PS Converter3/1
  Demux/5 -> Simulink-PS Converter5/1
  Demux/6 -> Simulink-PS Converter6/1
  connections:
  Six-Pulse Gate Multiplexer/RConn1 -- G/RConn1
  Simulink-PS Converter1/RConn1 -- Six-Pulse Gate Multiplexer/LConn1
  Simulink-PS Converter3/RConn1 -- Six-Pulse Gate Multiplexer/LConn3
  Simulink-PS Converter5/RConn1 -- Six-Pulse Gate Multiplexer/LConn5
  Simulink-PS Converter6/RConn1 -- Six-Pulse Gate Multiplexer/LConn6
  Simulink-PS Converter4/RConn1 -- Six-Pulse Gate Multiplexer/LConn4
  Simulink-PS Converter2/RConn1 -- Six-Pulse Gate Multiplexer/LConn2

== system IPMSM_velocity_control/Motor and Inverter/Sensing Vdc ==
  PS-Simulink Converter4 : nesl_utility/PS-Simulink Converter  PhysicalDomain=network_engine_domain  SubClassName=ps_output  LeftPortType=input  RightPortType=output  PseudoPeriodic=off  Frequencies=[]  Unit=V  AffineConversion=off
      settings: SourceProductName=Utilities
  Voltage Sensor : fl_lib/Electrical/Electrical Sensors/Voltage Sensor
      settings: SourceProductName=Foundation Library
  + : PMIOPort  Side=Left
  - : PMIOPort  Port=2  Side=Right
  tag scope: Vdc=global
  wires:
  PS-Simulink Converter4/1 -> [Vdc]
  connections:
  Voltage Sensor/LConn1 -- +/RConn1
  Voltage Sensor/RConn2 -- -/RConn1
  PS-Simulink Converter4/LConn1 -- Voltage Sensor/RConn1

== system IPMSM_velocity_control/Motor and Inverter/Sensing trq ==
  PS-Simulink Converter3 : nesl_utility/PS-Simulink Converter  PhysicalDomain=network_engine_domain  SubClassName=ps_output  LeftPortType=input  RightPortType=output  PseudoPeriodic=off  Frequencies=[]  Unit=N*m  AffineConversion=off
      settings: SourceProductName=Utilities
  Torque Sensor : fl_lib/Mechanical/Mechanical Sensors/Ideal Torque Sensor
      settings: SourceProductName=Foundation Library
  R : PMIOPort  Side=Left
  C : PMIOPort  Port=2  Side=Right
  tag scope: Tq_meas=global
  wires:
  PS-Simulink Converter3/1 -> [Tq_meas]
  connections:
  Torque Sensor/RConn1 -- C/RConn1
  Torque Sensor/RConn2 -- PS-Simulink Converter3/LConn1
  Torque Sensor/LConn1 -- R/RConn1

== system IPMSM_velocity_control/Motor and Inverter/Sensing w a ==
  MRRef : fl_lib/Mechanical/Rotational Elements/Mechanical Rotational Reference
      settings: SourceProductName=Foundation Library
  Motion Sensor : fl_lib/Mechanical/Mechanical Sensors/Ideal Rotational Motion Sensor  wrap_angle=simscape.enum.onoff.off  offset=0 deg
      settings: SourceProductName=Foundation Library
  PS-Simulink Converter1 : nesl_utility/PS-Simulink Converter  PhysicalDomain=network_engine_domain  SubClassName=ps_output  LeftPortType=input  RightPortType=output  PseudoPeriodic=off  Frequencies=[]  Unit=rad/s  AffineConversion=off
      settings: SourceProductName=Utilities
  PS-Simulink Converter2 : nesl_utility/PS-Simulink Converter  PhysicalDomain=network_engine_domain  SubClassName=ps_output  LeftPortType=input  RightPortType=output  PseudoPeriodic=off  Frequencies=[]  Unit=rad  AffineConversion=off
      settings: SourceProductName=Utilities
  R : PMIOPort  Side=Left
  w : PMIOPort  Port=2  Side=Right
  tag scope: a=global, w=global
  wires:
  PS-Simulink Converter1/1 -> [w]
  PS-Simulink Converter2/1 -> [a]
  connections:
  R/RConn1 -- Motion Sensor/LConn1
  Motion Sensor/RConn2 -- PS-Simulink Converter1/LConn1 -- w/RConn1
  MRRef/LConn1 -- Motion Sensor/RConn1
  Motion Sensor/RConn3 -- PS-Simulink Converter2/LConn1

== system IPMSM_velocity_control/Motor and Inverter/Sensing iabc ==
  Current Sensor : ee_lib/Sensors & Transducers/Current Sensor (Three-Phase)
      settings: SourceProductName=Electrical
  PS-Simulink Converter : nesl_utility/PS-Simulink Converter  PhysicalDomain=network_engine_domain  SubClassName=ps_output  LeftPortType=input  RightPortType=output  PseudoPeriodic=off  Frequencies=[]  Unit=A  AffineConversion=off
      settings: SourceProductName=Utilities
  1 : PMIOPort  Side=Left
  2 : PMIOPort  Port=2  Side=Right
  tag scope: iabc=global
  wires:
  PS-Simulink Converter/1 -> [iabc]
  connections:
  1/RConn1 -- Current Sensor/LConn1
  2/RConn1 -- Current Sensor/RConn2
  Current Sensor/RConn1 -- PS-Simulink Converter/LConn1

== system IPMSM_velocity_control/Motor and Inverter/TL = f(w^2,w) ==
  PS Add : fl_lib/Physical Signals/Functions/PS Add
  PS Gain1 : fl_ps_legacy_lib/Legacy Physical Signals/Functions/PS Gain  gain=1/300
  PS Math Function1 : fl_ps_legacy_lib/Legacy Physical Signals/Functions/PS Math Function  fcn_choice=7
      settings: SourceProductBaseCode=SS  InternalSimscapePortConfiguration="{\"Bottom\":[],\"Left\":[{\"id\":\"I\",\"label\":\"\",\"type\":\"input\"}],\"Right\":[{\"id\":\"O\",\"label\":\"\",\"type\":\"output\"}],\"Top\":[]}"
  load_torque1 : fl_ps_legacy_lib/Legacy Physical Signals/Functions/PS Gain  gain=-0.001584786820657
  load_torque2 : fl_ps_legacy_lib/Legacy Physical Signals/Functions/PS Gain  gain=-0.000001829134907
  w : PMIOPort  Side=Left
  TL : PMIOPort  Port=2  Side=Right
  connections:
  PS Math Function1/RConn1 -- load_torque2/LConn1
  PS Gain1/RConn1 -- load_torque1/LConn1 -- PS Math Function1/LConn1
  PS Gain1/LConn1 -- w/RConn1
  TL/RConn1 -- PS Add/RConn1
  PS Add/LConn1 -- load_torque1/RConn1
  PS Add/LConn2 -- load_torque2/RConn1

== system IPMSM_velocity_control/UDP_Communication/critical point filter  ==
  In1 : Inport
  Constant : Constant
  Constant1 : Constant  Value=0
  Enabled Subsystem : Subsystem  TreatAsAtomicUnit=on
  If : If  IfExpression=(u1 < 0.00001) & (u1 >-0.00001)
  If Action Subsystem : Subsystem  TreatAsAtomicUnit=on
  If Action Subsystem1 : Subsystem  TreatAsAtomicUnit=on
  Merge : Merge  InitialOutput=[0]
  Out_held : Outport
  wires:
  In1/1 -> Enabled Subsystem/1(In1), If/1
  If/1 -> If Action Subsystem/Action
  If/2 -> If Action Subsystem1/Action
  If Action Subsystem/1(Out1) -> Merge/1
  If Action Subsystem1/1(Out1) -> Merge/2
  Constant/1 -> If Action Subsystem1/1(In1)
  Constant1/1 -> If Action Subsystem/1(In1)
  Merge/1 -> Enabled Subsystem/Enable
  Enabled Subsystem/1(Out_without_filtering) -> Out_held/1

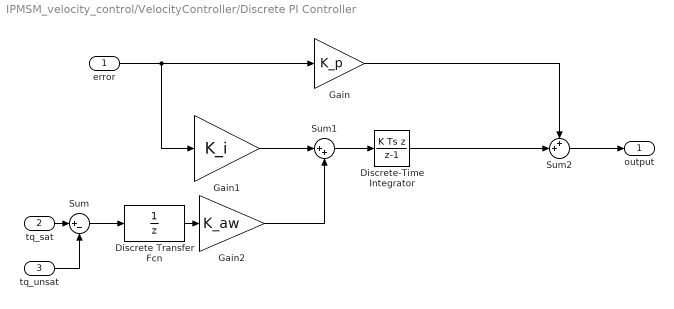
== system IPMSM_velocity_control/VelocityController/Discrete PI Controller ==
  error : Inport
  tq_sat : Inport  Port=2
  tq_unsat : Inport  Port=3
  Discrete Transfer Fcn : DiscreteTransferFcn  Denominator=[1 0]
  Discrete-Time Integrator : DiscreteIntegrator  IntegratorMethod=Integration: Backward Euler  SampleTime=msg_period  ICPrevOutput=DiscIntNeverNeededParam  ICPrevScaledInput=DiscIntNeverNeededParam
  Gain : Gain  Gain=K_p
  Gain1 : Gain  Gain=K_i
  Gain2 : Gain  Gain=K_aw
  Sum : Sum  Inputs=|+-
  Sum1 : Sum  Inputs=|++
  Sum2 : Sum  Inputs=++|
  output : Outport
  wires:
  error/1 -> Gain1/1, Gain/1
  Sum2/1 -> output/1
  Gain/1 -> Sum2/1
  Gain1/1 -> Sum1/1
  Sum1/1 -> Discrete-Time Integrator/1
  Discrete-Time Integrator/1 -> Sum2/2
  Discrete Transfer Fcn/1 -> Gain2/1
  Gain2/1 -> Sum1/2
  tq_sat/1 -> Sum/1
  Sum/1 -> Discrete Transfer Fcn/1
  tq_unsat/1 -> Sum/2

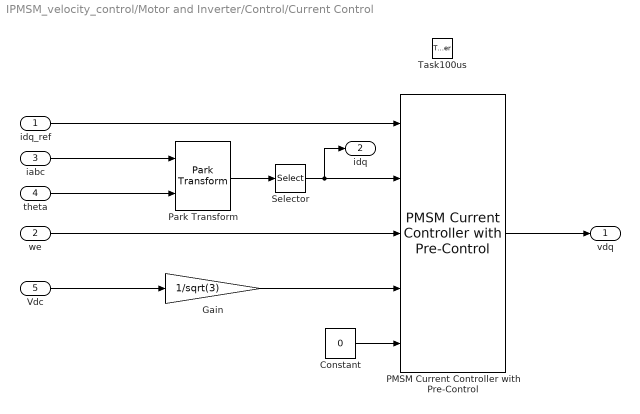
== system IPMSM_velocity_control/Motor and Inverter/Control/Current Control ==
  idq_ref : Inport
  we : Inport  Port=2
  iabc : Inport  Port=3
  theta : Inport  Port=4
  Vdc : Inport  Port=5
  Task100us : TriggerPort  TriggerType=function-call  VariantControl=Variant  PortDimensions=1
  Constant : Constant  Value=0  SampleTime=-1
  Gain : Gain  Gain=1/sqrt(3)
  PMSM Current Controller with Pre-Control : eePmsmCurrentController/PMSM Current Controller with Pre-Control  Kp_id=Kp_id  Ki_id=Ki_id  Kaw_id=1  Kp_iq=Kp_iq  Ki_iq=Ki_iq  Kaw_iq=1  Ts=-1  Tsd=Tsi  AxisPrio=Q-axis  ActZC=on  ActFF=on  idVect=[-200, 0, 200]  iqVect=[-200, 0, 200]  LdMatrix=Ld * ones(3, 3)  LqMatrix=Lq * ones(3, 3)  psimMatrix=psim * ones(3, 3)
      settings: SourceProductBaseCode=PS
  Park Transform : eeTransforms/Park Transform  AxisAlignment=Q-axis  PowerInvariant=off
  Selector : Selector  InputPortWidth=3  IndexOptions=Index vector (dialog)  Indices=[1 2]  OutputSizes=1
  vdq : Outport  VectorParamsAs1DForOutWhenUnconnected=off
  idq : Outport  Port=2  VectorParamsAs1DForOutWhenUnconnected=off
  wires:
  Park Transform/1 -> Selector/1
  Gain/1 -> PMSM Current Controller with Pre-Control/4
  Selector/1 -> idq/1, PMSM Current Controller with Pre-Control/2
  Constant/1 -> PMSM Current Controller with Pre-Control/5
  PMSM Current Controller with Pre-Control/1 -> vdq/1
  we/1 -> PMSM Current Controller with Pre-Control/3
  idq_ref/1 -> PMSM Current Controller with Pre-Control/1
  theta/1 -> Park Transform/2
  iabc/1 -> Park Transform/1
  Vdc/1 -> Gain/1

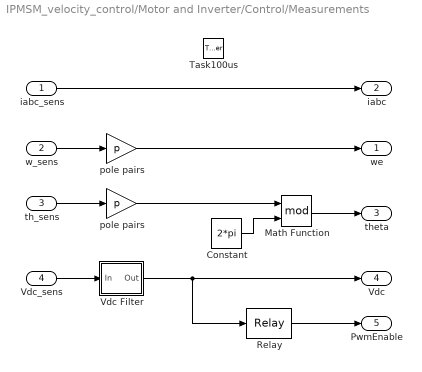
== system IPMSM_velocity_control/Motor and Inverter/Control/Measurements ==
  iabc_sens : Inport
  w_sens : Inport  Port=2
  th_sens : Inport  Port=3
  Vdc_sens : Inport  Port=4
  Task100us : TriggerPort  TriggerType=function-call  VariantControl=Variant  PortDimensions=1
  Constant : Constant  Value=2*pi  SampleTime=-1
  Math Function : Math  Operator=mod  SignedPower=on  SaturateOnIntegerOverflow=on
  Relay : Relay  OnSwitchValue=VDC_VECT(1)  OffSwitchValue=0.5*VDC_VECT(1)
  Vdc Filter : Subsystem  mask(Discrete first-order filter (Low-pass)){T=0.005, Ts=1e-4}
      mask prompts: T "Time constant (s):"; Ts "Sample time (s):"
      mask help: This block implements a discrete low-pass filter. To calculate the coefficients, the block discretises a continuous low-pass filter using the Tustin method.
      mask init:
      | num = [ Ts/(2*T + Ts), Ts/(2*T + Ts)];
      | den = [ 1, -(2*T - Ts)/(2*T + Ts)];
  pole pairs : Gain  Gain=p
  "pole pairs " : Gain  Gain=p
  we : Outport  VectorParamsAs1DForOutWhenUnconnected=off
  iabc : Outport  Port=2  VectorParamsAs1DForOutWhenUnconnected=off
  theta : Outport  Port=3  VectorParamsAs1DForOutWhenUnconnected=off
  Vdc : Outport  Port=4  VectorParamsAs1DForOutWhenUnconnected=off
  PwmEnable : Outport  Port=5  VectorParamsAs1DForOutWhenUnconnected=off
  wires:
  pole pairs/1 -> we/1
  Vdc_sens/1 -> Vdc Filter/1(In)
  th_sens/1 -> "pole pairs "/1
  w_sens/1 -> pole pairs/1
  iabc_sens/1 -> iabc/1
  "pole pairs "/1 -> Math Function/1
  Constant/1 -> Math Function/2
  Math Function/1 -> theta/1
  Relay/1 -> PwmEnable/1
  Vdc Filter/1(Out) -> Relay/1, Vdc/1

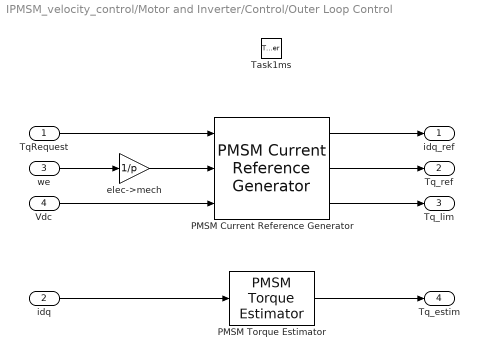
== system IPMSM_velocity_control/Motor and Inverter/Control/Outer Loop Control ==
  TqRequest : Inport
  idq : Inport  Port=2
  we : Inport  Port=3
  Vdc : Inport  Port=4
  Task1ms : TriggerPort  TriggerType=function-call  VariantControl=Variant  PortDimensions=1
  PMSM Current Reference Generator : eePmsmCurrentReferenceGen/PMSM Current Reference Generator  Vnom=Vnom  Pmax=Pmax  Tmax=Tmax  Ts=-1  RefType=Lookup-table based  rpmVec=RPM_VECT  TqVec=TQ_VECT  VdcVec=VDC_VECT  PWMMode=SVM: space vector modulation  ModFactor=1  idMatrix=ID_MAP  iqMatrix=IQ_MAP  p=8  psim=0.04  Ld=0.00024  Lq=0.00029  Rs=0.01  RefExpEnable=0
      settings: SourceProductBaseCode=PS
  PMSM Torque Estimator : eePmsmTorqueEstimator/PMSM Torque Estimator  ParamType=Constant parameters  p=p  idVect=[-200, 200]  iqVect=[-200, 200]  LdMatrix=0.0002 * ones(2, 2)  LqMatrix=0.0002 * ones(2, 2)  psimMatrix=0.04 * ones(2, 2)  Ld=Ld  Lq=Lq  psim=psim  Ts=-1
      settings: SourceProductBaseCode=PS
  elec->mech : Gain  Gain=1/p
  idq_ref : Outport  VectorParamsAs1DForOutWhenUnconnected=off
  Tq_ref : Outport  Port=2  VectorParamsAs1DForOutWhenUnconnected=off
  Tq_lim : Outport  Port=3  VectorParamsAs1DForOutWhenUnconnected=off
  Tq_estim : Outport  Port=4  VectorParamsAs1DForOutWhenUnconnected=off
  wires:
  we/1 -> elec->mech/1
  elec->mech/1 -> PMSM Current Reference Generator/2
  TqRequest/1 -> PMSM Current Reference Generator/1
  Vdc/1 -> PMSM Current Reference Generator/3
  PMSM Current Reference Generator/1 -> idq_ref/1
  PMSM Current Reference Generator/2 -> Tq_ref/1
  PMSM Current Reference Generator/3 -> Tq_lim/1
  idq/1 -> PMSM Torque Estimator/1
  PMSM Torque Estimator/1 -> Tq_estim/1

== system IPMSM_velocity_control/UDP_Communication/critical point filter /Enabled Subsystem ==
  In1 : Inport
  Enable : EnablePort
  Out_without_filtering : Outport
  wires:
  In1/1 -> Out_without_filtering/1

== system IPMSM_velocity_control/UDP_Communication/critical point filter /If Action Subsystem ==
  In1 : Inport
  Action Port : ActionPort
  Out1 : Outport
  wires:
  In1/1 -> Out1/1

== system IPMSM_velocity_control/UDP_Communication/critical point filter /If Action Subsystem1 ==
  In1 : Inport
  Action Port : ActionPort
  Out1 : Outport
  wires:
  In1/1 -> Out1/1

== system IPMSM_velocity_control/Motor and Inverter/Control/Measurements/Vdc Filter ==
  In : Inport
  Discrete Transfer Fcn : DiscreteTransferFcn  Numerator=num  Denominator=den
  Out : Outport  VectorParamsAs1DForOutWhenUnconnected=off
  wires:
  Discrete Transfer Fcn/1 -> Out/1
  In/1 -> Discrete Transfer Fcn/1

== stateflow chart IPMSM_velocity_control/Motor and Inverter/Control/Task Scheduler ==
  (default) -> (junction 23) : CLK_50us
  (junction 23) -> (junction 17)
  (junction 17) -> (junction 22) [order 2]
  (junction 17) -> (junction 22) [order 1] : [cnt%%2==0]{Task_100us_1;}
  (junction 22) -> (junction 18) [order 2]
  (junction 22) -> (junction 18) [order 1] : [cnt%%2==0]{Task_100us_2;}
  (junction 18) -> (junction 21) [order 1] : [cnt%%20==0]{Task_1ms_1;}
  (junction 18) -> (junction 21) [order 2]
  (junction 21) -> (junction 34) [order 2]
  (junction 21) -> (junction 16) [order 1] : [1]{cnt++;}
  data: cnt local int32
  events: Task_100us_1 output FUNCTION_CALL_EVENT; Task_100us_2 output FUNCTION_CALL_EVENT; Task_1ms_1 output FUNCTION_CALL_EVENT; CLK_50us input FUNCTION_CALL_EVENT

== matlab function IPMSM_velocity_control/Messages_to_send/Message_Control/MATLAB Function ==
  data: u input; y output

function y = fcn(u)

persistent id_select;

if isempty(id_select)
    id_select = 1;
end
%tempo de transição para enviar frames de mesmo período
can_delay = 0.5e-3;
%tempo da simulação
time = u;
%periodos de envio de cada classe de mensagem

%mensagens com periodo de 10ms
analog_input_voltages_period = 10e-3;
digital_input_status_period = 10e-3;
motor_position_period = 10e-3;
current_information_period = 10e-3;
voltage_information_period = 10e-3;
flux_information_period = 10e-3;
internal_states_period = 10e-3;
torque_and_timer_info_period = 10e-3;
modu_indexand_flux_weakening_out_period  = 10e-3;

%mensagens com periodo de 100ms
temperatures1_period = 100e-3;
temperatures2_period = 100e-3;
temperatures3_period = 100e-3;
internal_voltages_period = 100e-3;
fault_codes_period = 100e-3;
firmware_info_period = 100e-3;

%verifica primeiro todas as mensagens de periodo = 10ms
if rem(time - 1*can_delay,analog_input_voltages_period) == 0
    id_select = 1;
elseif rem(time - 2*can_delay,digital_input_status_period) == 0
    id_select = 2;
elseif rem(time - 3*can_delay,motor_position_period) == 0
    id_select = 3;
elseif rem(time - 4*can_delay,current_information_period) == 0
    id_select = 4;
elseif rem(time - 5*can_delay,voltage_information_period) == 0
    id_select = 5; 
elseif rem(time - 6*can_delay,flux_information_period) == 0
    id_select = 6;
elseif rem(time - 7*can_delay,internal_states_period) == 0
    id_select = 7; 
elseif rem(time - 8*can_delay,torque_and_timer_info_period) == 0
    id_select = 8; 
elseif rem(time - 9*can_delay,modu_indexand_flux_weakening_out_period)== 0
    id_select = 9; 
    
%verifica as mensagens com periodo de 100ms
elseif rem(time - 10*can_delay,temperatures1_period)== 0
    id_select = 10;
elseif rem(time - 11*can_delay,temperatures2_period)== 0
    id_select = 11;
elseif rem(time - 12*can_delay,temperatures3_period)== 0
    id_select = 12;
elseif rem(time - 13*can_delay,internal_voltages_period)== 0
    id_select = 13;
elseif rem(time - 14*can_delay,fault_codes_period)== 0
    id_select = 14;
elseif rem(time - 15*can_delay,firmware_info_period)== 0
    id_select = 15;    
end
y = id_select;
